simulink library "sm_worm_jack_lib"  (R2021b)
settings: Solver=VariableStepAuto  StartTime=0.0  StopTime=10.0  RelTol=1e-3
undefined symbols (not defined in the file or in its folder): Hand, Right, X, Y, Z
libraries: sm_lib x37, $bdroot x11, nesl_utility x8
(part 1 of 2)
settings Model: Creator=The MathWorks, Inc.  LastModifiedBy=The MathWorks, Inc.
settings SolverCC: AlgebraicLoopSolver=TrustRegion
settings DataIOCC: ReturnWorkspaceOutputs=off
settings DebuggingCC: SFMachineParentedDataDiag=warning  ArithmeticOperatorsInVariantConditions=warning
settings SFSimCC: SimUseLocalCustomCode=off  CustomCodeUndefinedFunction=UseInterfaceOnly
settings RTWCC: RTWUseLocalCustomCode=off
settings CodeAppCC: StateflowObjectComments=on

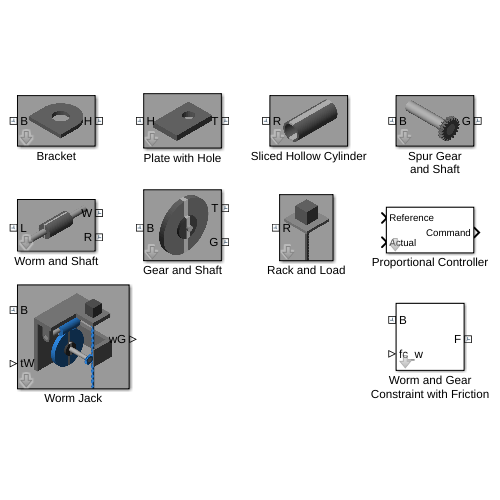
[thumbnail: Simulink's stored preview of the top-level diagram]
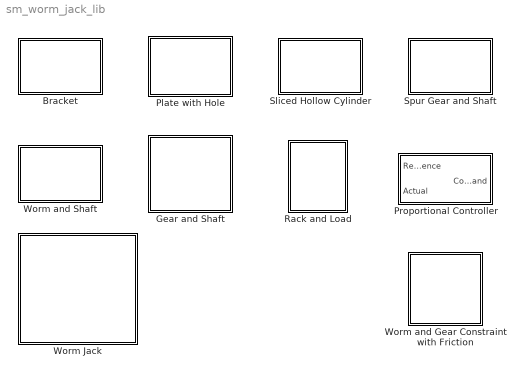
== system sm_worm_jack_lib ==
  Bracket : Subsystem  mask(Bracket){height=0.1, width=0.1, thickness=0.01, holeOffset=0.05, holeRadius=0.02, rho=2700, color=[0.5 0.5 0.5]}
      mask prompts: height "Height (m)"; width "Width (m)"; thickness "Thickness (m)"; holeOffset "Hole Offset (m)"; holeRadius "Hole Radius (m)"; rho "Density (kg/m^3)"; color "Color [r g b]"
      mask help:
      | This block models a bracket.
      |
      | Port B corresponds to the center point on the base face. Port H corresponds to the center of the hole.
      mask init:
      | points = 40;
      | 
      | y = height - 0.5*width;
      | 
      | outerVertices = ...
      |   [          0      0;...
      |      0.5*width      0;...
      |      0.5*width      y;...
      |      0.5*width height;...
      |     -0.5*width height;...
      |     -0.5*width      y;...
      |     -0.5*width      0;...
      |              0      0];
      | 
      | outer = simmechanics.demohelpers.round_corners(...
      |   outerVertices, [4 5], 0.5*width, points);
      | 
      | holeTheta = linspace(1.5*pi, -0.5*pi, points);
      | 
      | hole = [holeRadius*cos(holeTheta);...
      |         holeRadius*sin(holeTheta)+holeOffset]';
      | 
      | crossSection = [hole; outer];
      mask DialogControl Tab1 Prompt: Dimensions
      mask DialogControl Tab2 Prompt: Material Properties
      mask Display:
      | image(fullfile(matlabroot,'toolbox','physmod','sm','smdemos','worm_jack','images','sm_worm_jack_bracket.png'));
      | port_label('lconn',1,'B');
      | port_label('rconn',1,'H');
  Gear and Shaft : Subsystem  mask(Gear and Shaft){gearRadius=0.1, gearLength=0.02, shaftRadius=0.01, shaftLength=0.1, collarRadius=0.04, gearOffset=0.02, rhoGear=2700, rhoShaft=2700, rhoCollar=2700, gearColor=[0.5 0.5 0.5], shaftColor=[0.8 0.8 0.8], collarColor=[0.3 0.3 0.3], sliceColor=[0.9 0.9 0.9]}
      mask prompts: gearRadius "Gear Radius (m)"; gearLength "Gear Length (m)"; shaftRadius "Shaft Radius (m)"; shaftLength "Shaft Length (m)"; collarRadius "Collar Radius (m)"; gearOffset "Axial Offset (m)"; rhoGear "Gear Density (kg/m^3)"; rhoShaft "Shaft Density (kg/m^3)"; rhoCollar "Collar Density (kg/m^3)"; gearColor "Gear Color [r g b]"; shaftColor "Shaft Color [r g b]"; collarColor "Collar Color [r g b]"; sliceColor "Slice Color [r g b]"
      mask help:
      | This block models a gear mounted on a shaft with a collar. The gear, collar and shaft are concentric and the axial distance between the gear's midpoint and the shaft's midpoint can be adjusted.
      |
      | Ports B and T correspond to center points on the bottom and top faces of the shaft, respectively. Port G corresponds to the center of the gear.
      mask init:
      | offsetFromTop = 0.5*shaftLength-gearOffset;
      | 
      | sliceThickness = 0.4*collarRadius;
      mask DialogControl Tab1 Prompt: Dimensions
      mask DialogControl Tab2 Prompt: Material Properties
      mask Display:
      | image(fullfile(matlabroot,'toolbox','physmod','sm','smdemos','worm_jack','images','sm_worm_jack_gearshaft.png'));
      | port_label('lconn',1,'B');
      | port_label('rconn',1,'T');
      | port_label('rconn',2,'G');
  Plate with Hole : Subsystem  mask(Plate with Hole){height=0.15, width=0.1, thickness=0.02, holeRadius=0.02, holeOffset=0.1, rho=2700, color=[0.5 0.5 0.5]}
      mask prompts: height "Height (m)"; width "Width (m)"; thickness "Thickness (m)"; holeRadius "Hole Radius (m)"; holeOffset "Hole Offset (m)"; rho "Density (kg/m^3)"; color "Color [r g b]"
      mask help:
      | This block models a plate with a hole. The center of the hole is on the plate's longitudinal axis.
      |
      | Port H corresponds to the center of the hole. Port T corresponds to the center point on the top rear edge.
      mask init:
      | points = 40;
      | 
      | y = height - 0.5*width;
      | 
      | outer = ...
      |   [          0      0;...
      |      0.5*width      0;...
      |      0.5*width      y;...
      |      0.5*width height;...
      |     -0.5*width height;...
      |     -0.5*width      y;...
      |     -0.5*width      0;...
      |              0      0];
      | 
      | holeTheta = linspace(1.5*pi, -0.5*pi, points);
      | 
      | hole = [holeRadius*cos(holeTheta);...
      |         holeRadius*sin(holeTheta)+holeOffset]';
      | 
      | crossSection = [hole; outer];
      mask DialogControl Tab1 Prompt: Dimensions
      mask DialogControl Tab2 Prompt: Material Properties
      mask Display:
      | image(fullfile(matlabroot,'toolbox','physmod','sm','smdemos','worm_jack','images','sm_worm_jack_platehole.png'));
      | port_label('lconn',1,'H');
      | port_label('rconn',1,'T');
  Proportional Controller : Subsystem  mask(PID Controller){Kp=1}
      mask help:
      | This block models a proportional controller using Simulink blocks.
      |
      | This block takes in a reference signal and actual signal to calculate a control command.
  Rack and Load : Subsystem  mask(Rack and Load){rackWidth=0.01, rackBase=0.005, toothPitch=0.006, rackLength=0.3, plateWidth=0.1, plateThickness=0.01, loadWidth=0.05, rackRho=2700, plateRho=2700, loadRho=2700, rackColor=[0.5 0.5 0.5], plateColor=[0.7 0.7 0.7], loadColor=[0.5 0.5 0.5]}
      mask prompts: rackWidth "Rack Width (m)"; rackBase "Rack Base Thickness (m)"; toothPitch "Tooth Pitch (m)"; rackLength "Rack Length (m)"; plateWidth "Plate Width (m)"; plateThickness "Plate Thickness (m)"; loadWidth "Load Width (m)"; rackRho "Rack Density (kg/m^3)"; plateRho "Plate Density (kg/m^3)"; loadRho "Load Density (kg/m^3)"; rackColor "Rack Color [r g b]"; plateColor "Plate Color [r g b]"; loadColor "Load Color [r g b]"
      mask help:
      | This block models a rack that is attached to a load. The load consists of a brick which is carried on a rectangular plate.
      |
      | Port R corresponds to the center of the rack.
      mask init:
      | plateDimensions = [plateWidth plateWidth plateThickness];
      | loadDimensions  = loadWidth*[1 1 1];
      | 
      | numTeeth = ceil(rackLength/toothPitch);
      | 
      | rackCrossSection = ...
      |   simmechanics.demohelpers.rack_profile(toothPitch,numTeeth,rackBase);
      mask DialogControl TabVar1 Prompt: Dimensions
      mask DialogControl TabVar2 Prompt: Material Properties
      mask Display:
      | image(fullfile(matlabroot,'toolbox','physmod','sm','smdemos','worm_jack','images','sm_worm_jack_rackload.png'));
      | port_label('lconn',1,'R');
  Sliced Hollow Cylinder : Subsystem  mask(Sliced Hollow Cylinder){outerRadius=0.1, innerRadius=0.09, length=0.5, sliceThickness=0.06, rho=2700, mainColor=[0.5 0.5 0.5], sliceColor=[0.9 0.9 0.9]}
      mask prompts: outerRadius "Outer Radius (m)"; innerRadius "Inner Radius (m)"; length "Length (m)"; sliceThickness "Slice Thickness (m)"; rho "Density (kg/m^3)"; mainColor "Main Color [r g b]"; sliceColor "Slice Color [r g b]"
      mask help:
      | This block models a hollow cylinder where a slice of the cylinder can be set to a different color.
      |
      | Port R corresponds to the center of the cylinder.
      mask init:
      | points = 30;
      | 
      | outerTheta = acos(0.5*sliceThickness / outerRadius);
      | 
      | rightOuterThetaVect = linspace(  -outerTheta,      outerTheta, points);
      | leftOuterThetaVect  = linspace(pi-outerTheta,   pi+outerTheta, points);
      | topOuterThetaVect   = linspace(   outerTheta,   pi-outerTheta, points);
      | botOuterThetaVect   = linspace(pi+outerTheta, 2*pi-outerTheta, points);
      | 
      | if (sliceThickness > 2*innerRadius)
      |   % The slice is wider than the hole
      |   rightCrossSection = [outerRadius*cos(rightOuterThetaVect);...
      |                        outerRadius*sin(rightOuterThetaVect)]';
      |   leftCrossSection  = [outerRadius*cos(leftOuterThetaVect);...
      |                        outerRadius*sin(leftOuterThetaVect)]';
      | 
      |   topInnerThetaVect = linspace(pi, 0, points);
      |   botInnerThetaVect = linspace(0, -pi, points);
      |   
      |   topCrossSection = [...
      |     outerRadius*cos(topOuterThetaVect) -0.5*sliceThickness innerRadius*cos(topInnerThetaVect) 0.5*sliceThickness;...
      |     outerRadius*sin(topOuterThetaVect) 0 innerRadius*sin(topInnerThetaVect) 0]';
      |   
      |   botCrossSection = [...
      |     outerRadius*cos(botOuterThetaVect) 0.5*sliceThickness innerRadius*cos(botInnerThetaVect) -0.5*sliceThickness;...
      |     outerRadius*sin(botOuterThetaVect) 0 innerRadius*sin(botInnerThetaVect) 0]';
      | else
      |   % The slicer is narrower than the hole
      |   innerTheta = acos(0.5*sliceThickness / innerRadius);
      |   
      |   rightInnerThetaVect = linspace(   innerTheta,    -innerTheta, points);
      |   leftInnerThetaVect  = linspace(pi+innerTheta,  pi-innerTheta, points);
      |   topInnerThetaVect   = linspace(pi-innerTheta,     innerTheta, points);
      |   botInnerThetaVect   = linspace(  -innerTheta, -pi+innerTheta, points);
      |   
      |   rightCrossSection = [...
      |     outerRadius*cos(rightOuterThetaVect) innerRadius*cos(rightInnerThetaVect);...
      |     outerRadius*sin(rightOuterThetaVect) innerRadius*sin(rightInnerThetaVect)]';
      |   leftCrossSection  = [...
      |     outerRadius*cos(leftOuterThetaVect)  innerRadius*cos(leftInnerThetaVect);...
      |     outerRadius*sin(leftOuterThetaVect)  innerRadius*sin(leftInnerThetaVect)]';
      |   topCrossSection   = [...
      |     outerRadius*cos(topOuterThetaVect)   innerRadius*cos(topInnerThetaVect);...
      |     outerRadius*sin(topOuterThetaVect)   innerRadius*sin(topInnerThetaVect)]';
      |   botCrossSection   = [...
      |     outerRadius*cos(botOuterThetaVect)   innerRadius*cos(botInnerThetaVect);...
      |     outerRadius*sin(botOuterThetaVect)   innerRadius*sin(botInnerThetaVect)]';
      | end
      mask DialogControl Tab1 Prompt: Dimensions
      mask DialogControl Tab2 Prompt: Material Properties
      mask Display:
      | image(fullfile(matlabroot,'toolbox','physmod','sm','smdemos','worm_jack','images','sm_worm_jack_slicedhollowcylinder.png'));
      | port_label('lconn',1,'R');
  Spur Gear and Shaft : Subsystem  mask(Pinion Gear and Shaft){gearRadius=0.02, numTeeth=20, gearLength=0.01, shaftRadius=0.01, shaftLength=0.1, gearRho=2700, shaftRho=2700, gearColor=[0.5 0.5 0.5], shaftColor=[0.8 0.8 0.8]}
      mask prompts: gearRadius "Gear Radius (m)"; numTeeth "Number of Teeth"; gearLength "Gear Length (m)"; shaftRadius "Shaft Radius (m)"; shaftLength "Shaft Length (m)"; gearRho "Gear Density (kg/m^3)"; shaftRho "Shaft Density (kg/m^3)"; gearColor "Gear Color [r g b]"; shaftColor "Shaft Color [r g b]"
      mask help:
      | This block models a spur gear on a shaft. The gear and shaft are concentric and the number of gear teeth can be adjusted.
      |
      | Port B corresponds to the center point on the bottom face of the shaft. Port G corresponds to the center of the gear.
      mask init:
      | gearCrossSection = simmechanics.demohelpers.gear_profile(2*gearRadius,numTeeth);
      | gearCrossSection = [gearCrossSection; gearCrossSection(1,:)];
      | 
      | th = linspace(0,-2*pi,100)';
      | holeCrossSection = [shaftRadius*cos(th) shaftRadius*sin(th)];
      | 
      | gearCrossSection = [gearCrossSection; holeCrossSection];
      mask DialogControl TabVar1 Prompt: Dimensions
      mask DialogControl TabVar2 Prompt: Material Properties
      mask Display:
      | image(fullfile(matlabroot,'toolbox','physmod','sm','smdemos','worm_jack','images','sm_worm_jack_spurgearshaft.png'));
      | port_label('lconn',1,'B');
      | port_label('rconn',1,'G');
  Worm Jack : Subsystem  mask(Worm Drive Assembly){wormLeadAngle=10, wormRadius=0.025, wormLength=0.1, wormShaftLength=0.2, gearRadius=0.085, gearLength=0.02, gearShaftLength=0.1, collarRadius=0.03, shaftRadius=0.01, rackLength=0.4, pinionRadius=0.02, pinionTeeth=20, pinionShaftLength=0.1, loadWidth=0.05, plateThickness=0.02, wG_0=80, muK=0.5, muS=0.5, vth=1e-4, t_c=1e-6, wormRho=2700, gearRho=2700, shaftRho=2700, collarRho=2700, rackRho=2700, pinionRho=2700, housingRho=2700, boxRho=7800, wormColor=[0.2 0.6 1.0], gearColor=[0.2 0.6 1.0], shaftColor=[0.8 0.8 0.8], collarColor=[0.3 0.3 0.3], rackColor=[0.2 0.6 1.0], pinionColor=[0.2 0.6 1.0], housingColor=[0.6 0.6 0.6], boxColor=[0.4 0.4 0.4], sliceColor=[0.9 0.9 0.9]}
      mask prompts: wormLeadAngle "Worm Lead Angle (deg)"; wormRadius "Worm Radius (m)"; wormLength "Worm Length (m)"; wormShaftLength "Worm Shaft Length (m)"; gearRadius "Gear Radius (m)"; gearLength "Gear Length (m)"; gearShaftLength "Gear Shaft Length (m)"; collarRadius "Gear Collar Radius (m)"; shaftRadius "Shaft Radii (m)"; rackLength "Rack Length (m)"; pinionRadius "Pinion Radius (m)"; pinionTeeth "Pinion Teeth Number"; pinionShaftLength "Pinion Shaft Length (m)"; loadWidth "Load Width (m)"; plateThickness "Housing Plate Thickness (m)"; wG_0 "Initial Gear Revolute Velocity (deg/s)"; muK "Kinetic Friction Coefficient"; muS "Static Friction Coefficient"; vth "Velocity Threshold (m/s)"; t_c "Constraint Force Filter Constant (s)"; wormRho "Worm Density (kg/m^3)"; gearRho "Gear Density (kg/m^3)"; shaftRho "Shaft Density (kg/m^3)"; collarRho "Collar Density (kg/m^3)"; rackRho "Rack Density (kg/m^3)"; pinionRho "Pinion Density (kg/m^3)"; housingRho "Housing Density (kg/m^3)"; boxRho "Box Density (kg/m^3)"; wormColor "Worm Color [r g b]"; gearColor "Gear Color [r g b]"; shaftColor "Shaft Color [r g b]"; collarColor "Collar Color [r g b]"; rackColor "Rack Color [r g b]"; pinionColor "Pinion Color [r g b]"; housingColor "Housing Color [r g b]"; boxColor "Box Color [r g b]"; sliceColor "Slice Color [r g b]"
      mask help:
      | This block models a worm jack. The mechanism consists of a worm drive coupled to a rack and pinion.
      |
      | Port B corresponds to the center of the hole where the gear shaft is mounted.
      |
      | The input port tW specifies the torque input to the worm revolute joint. Output port wG corresponds to the angular velocity of the gear revolute joint.
      mask init:
      | wormShaftLength   = 2*gearRadius + 4*plateThickness;
      | pinionLength      = 0.5*pinionRadius;
      | rackWidth         = pinionLength;
      | rackBase          = 0.5*pinionLength;
      | toothPitch        = 2*pi*pinionRadius/pinionTeeth;
      | gearOffset        = 0.5*(gearShaftLength-3*gearLength);
      | housingHoleRadius = 1.1*shaftRadius;
      | gearSupHeight     = 2*gearRadius + 2*wormRadius + plateThickness;
      | bracketHoleOffset = plateThickness + wormRadius;
      | bracketHoleRadius = housingHoleRadius;
      | bracketWidth      = 4*shaftRadius;
      | bracketHeight     = bracketHoleOffset + 0.5*bracketWidth;
      | 
      | wormSupportDims = [wormShaftLength plateThickness gearShaftLength];
      | 
      | leftBracketOffset   = [ 0.5*(plateThickness-wormShaftLength) ...
      |                        -0.5*plateThickness                   ...
      |                         0.5*gearShaftLength-1.5*gearLength];
      |                       
      | rightBracketOffset  = [ 0.5*(wormShaftLength-plateThickness) ...
      |                        -0.5*plateThickness                   ...
      |                         0.5*gearShaftLength-1.5*gearLength];
      | 
      | % Rack Support
      | 
      | sidePlateYDim = (gearShaftLength+pinionShaftLength-1.5*plateThickness-0.5*pinionLength);
      | sidePlateDim  = [gearRadius sidePlateYDim plateThickness];
      | 
      | frontPlateYDim = (0.5*wormShaftLength-2*pinionRadius);
      | frontPlateDim  = [gearRadius frontPlateYDim plateThickness];
      | 
      | rackSupportOffset   = [0.5*(wormShaftLength-plateThickness) ...
      |                        0                                    ...
      |                        0.5*plateThickness];
      | 
      | guideDepth = pinionRadius;
      | guideWidth = pinionRadius;
      | 
      | guideCrossSection = [-0.5 *guideWidth 0;              ...
      |                       0.5 *guideWidth 0;              ...
      |                       0.5 *guideWidth guideDepth;     ...
      |                       0.25*guideWidth guideDepth;     ...
      |                       0.25*guideWidth 0.5*guideDepth; ...
      |                      -0.25*guideWidth 0.5*guideDepth; ...
      |                      -0.25*guideWidth guideDepth;     ...
      |                      -0.5 *guideWidth guideDepth];
      mask DialogControl Tab1 Prompt: Dimensions
      mask DialogControl Tab2 Prompt: Internal Mechanics
      mask DialogControl Tab3 Prompt: Material Properties
      mask Display:
      | image(fullfile(matlabroot,'toolbox','physmod','sm','smdemos','worm_jack','images','sm_worm_jack_wormjack.png'));
      | port_label('lconn',1,'B');
      | port_label('lconn',2,'tW');
      | port_label('rconn',1,'wG');
  Worm and Gear Constraint with Friction : Subsystem  mask(Worm and Gear Constraint with Friction){wormDirection=Right-Hand, wormLeadAngle=10, wormRadius=0.025, gearRadius=0.085, frictionToggle=on, muK=0.5, muS=0.5, vth=1e-4, t_c=1e-6}
      mask prompts: wormDirection "Worm Direction"; wormLeadAngle "Worm Lead Angle (deg)"; wormRadius "Worm Radius (m)"; gearRadius "Gear Radius (m)"; frictionToggle "Enable Friction"; muK "Kinetic Friction Coefficient"; muS "Static Friction Coefficient"; vth "Sliding Velocity Threshold (m/s)"; t_c "Constraint Force Filter Constant (s)"
      mask help:
      | This block models a Worm and Gear Constraint with friction. The worm rotates about the base z-axis and the gear rotates about the follower z-axis.
      |
      | Ports B and F are frame ports that represent the base and follower frames of the Worm and Gear Constraint block, respectively. The constraint force signal from the worm's revolute joint must be provided through port fc_w.
      mask init:
      | blockPath = gcb;
      | wgcPath = [blockPath '/Worm and Gear Constraint'];
      | 
      | if wormDirection == 1
      |     set_param(wgcPath,'WormDirection','RightHand');
      |     wormDirGain = 1;
      | else
      |     set_param(wgcPath,'WormDirection','LeftHand');
      |     wormDirGain = -1;
      | end
      | 
      | if frictionToggle
      |     frcGain = 1;
      | else
      |     frcGain = 0;
      | end
      mask TypeOptions wormDirection: Right-Hand | Left-Hand
      mask DialogControl Tab1 Prompt: Properties
      mask DialogControl Tab2 Prompt: Internal Mechanics
  Worm and Shaft : Subsystem  mask(Worm and Shaft){wormRadius=0.025, wormLength=0.1, shaftRadius=0.01, shaftLength=0.25, rhoWorm=2700, rhoShaft=2700, wormColor=[0.5 0.5 0.5], shaftColor=[0.8 0.8 0.8], sliceColor=[0.9 0.9 0.9]}
      mask prompts: wormRadius "Worm Radius (m)"; wormLength "Worm Length (m)"; shaftRadius "Shaft Radius (m)"; shaftLength "Shaft Length (m)"; rhoWorm "Worm Density (kg/m^3)"; rhoShaft "Shaft Density (kg/m^3)"; wormColor "Worm Color [r g b]"; shaftColor "Shaft Color [r g b]"; sliceColor "Slice Color [r g b]"
      mask help:
      | This block models a worm mounted on a shaft. The worm and shaft are concentric and the worm is axially located at the midpoint of the shaft.
      |
      | Ports L and R correspond to center points on the left and right faces of the shaft, respectively. Port W corresponds to the center of the worm.
      mask init:
      | sliceThickness = 0.2*wormRadius;
      mask DialogControl Tab1 Prompt: Dimensions
      mask DialogControl Tab2 Prompt: Material Properties
      mask Display:
      | image(fullfile(matlabroot,'toolbox','physmod','sm','smdemos','worm_jack','images','sm_worm_jack_wormshaft.png'));
      | port_label('lconn',1,'L');
      | port_label('rconn',1,'W');
      | port_label('rconn',2,'R');

== system sm_worm_jack_lib/Bracket ==
  Bracket : sm_lib/Body Elements/Extruded Solid  GraphicAmbientColor=[0.15 0.15 0.15 1.0]  BasedOnType=Density  CenterOfMass=[0 0 0]  CenterOfMassUnits=m  GraphicDiffuseColor=color  ExportConvexHullGeometry=off  ExtrusionCrossSection=crossSection  ExtrusionCrossSectionUnits=m  Density=rho  DensityUnits=kg/m^3  DoExposeReferenceFrame=on  GraphicEmissiveColor=[0.0 0.0 0.0 1.0]  ExportEntireGeometry=off  ExtrusionLength=thickness  ExtrusionLengthUnits=m  ExtrusionType=General  SerializedFrames=<Frames/>  MarkerShape=Sphere  MarkerSize=10  GraphicType=FromGeometry  InertiaType=CalculateFromGeometry  Mass=1  MassUnits=kg  MomentsOfInertia=[1 1 1]  MomentsOfInertiaUnits=kg*m^2  PolygonNumSides=3  GraphicOpacity=1.0  PolygonOuterRadius=1  PolygonOuterRadiusUnits=m  ProductsOfInertia=[1 1 1]  ProductsOfInertiaUnits=kg*m^2  GraphicShininess=75  GraphicSpecularColor=[0.5 0.5 0.5 1.0]  GraphicVisPropType=SimpleVisualProperties
  Hole xForm : sm_lib/Frames and Transforms/Rigid Transform  TranslationMethod=StandardAxis  TranslationStandardOffset=holeOffset  TranslationLengthUnit=m  TranslationStandardAxis=+Y  TranslationCartesianOffset=[0 0 0]  TranslationROffset=0  TranslationROffsetUnits=m  TranslationZOffset=0  TranslationZOffsetUnits=m  TranslationThetaOffset=0  TranslationThetaOffsetUnits=deg  RotationMethod=None  RotationAngleUnits=deg  RotationStandardAxis=+Y  RotationAngle=0.0  RotationArbitraryAxis=[0 0 1]  FollAlignAxisA=+X  BaseAlignAxisA=+Y  FollAlignAxisB=+Y  BaseAlignAxisB=+Z  RotationSequenceAxes=FollowerAxes  RotationSequence=XYX  RotationSequenceAngles=[0 0 0]  RotationSequenceAnglesUnits=deg  RotationMatrix=[1 0 0; 0 1 0; 0 0 1]
  B : PMIOPort  Side=Left
  H : PMIOPort  Port=2  Side=Right
  connections:
  B/RConn1 -- Hole xForm/LConn1 -- Bracket/RConn1
  H/RConn1 -- Hole xForm/RConn1

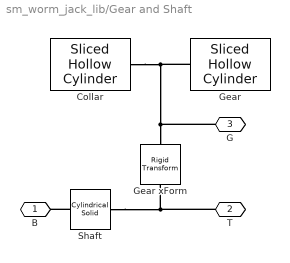
== system sm_worm_jack_lib/Gear and Shaft ==
  Collar : $bdroot/Sliced Hollow Cylinder  outerRadius=collarRadius  innerRadius=shaftRadius  length=2*gearLength  sliceThickness=sliceThickness  rho=rhoCollar  mainColor=collarColor  sliceColor=sliceColor
  Gear : $bdroot/Sliced Hollow Cylinder  outerRadius=gearRadius  innerRadius=collarRadius  length=gearLength  sliceThickness=sliceThickness  rho=rhoGear  mainColor=gearColor  sliceColor=sliceColor
  Gear xForm : sm_lib/Frames and Transforms/Rigid Transform  TranslationMethod=StandardAxis  TranslationStandardOffset=offsetFromTop  TranslationLengthUnit=m  TranslationStandardAxis=-Z  TranslationCartesianOffset=[0 0 0]  TranslationROffset=0  TranslationROffsetUnits=m  TranslationZOffset=0  TranslationZOffsetUnits=m  TranslationThetaOffset=0  TranslationThetaOffsetUnits=deg  RotationMethod=None  RotationAngleUnits=deg  RotationStandardAxis=+Z  RotationAngle=0.0  RotationArbitraryAxis=[0 0 1]  FollAlignAxisA=+X  BaseAlignAxisA=+Y  FollAlignAxisB=+Y  BaseAlignAxisB=+Z  RotationSequenceAxes=FollowerAxes  RotationSequence=XYX  RotationSequenceAngles=[0 0 0]  RotationSequenceAnglesUnits=deg  RotationMatrix=[1 0 0; 0 1 0; 0 0 1]
  Shaft : sm_lib/Body Elements/Cylindrical Solid  GraphicAmbientColor=[0.15 0.15 0.15 1.0]  BasedOnType=Density  CenterOfMass=[0 0 0]  CenterOfMassUnits=m  GraphicDiffuseColor=shaftColor  CylinderLength=shaftLength  CylinderLengthUnits=m  CylinderRadius=shaftRadius  CylinderRadiusUnits=m  Density=rhoShaft  DensityUnits=kg/m^3  DoExposeReferenceFrame=off  GraphicEmissiveColor=[0.0 0.0 0.0 1.0]  ExportEntireGeometry=off  SerializedFrames=<Frames><Frame><Id>Frame1</Id><Value><Name>T</Name><Origin><Source>GeometricFeature</Source><FeatureName>top surface</FeatureName></Origin><PrimaryAxis><DefinedDirection>+Z</DefinedDirection><Source>ReferenceFrame</Source><SourceDirection>+Z</SourceDirection><FeatureName></FeatureName></PrimaryAxis><SecondaryAxis><DefinedDirection>+X</DefinedDirection><Source>ReferenceFrame</Source><SourceDirection>+X</SourceDirection><FeatureName></FeatureName></SecondaryAxis></Value></Frame><Frame><Id>Frame2</Id><Value><Name>B</Name><Origin><Source>GeometricFeature</Source><FeatureName>bottom surface</FeatureName></Origin><PrimaryAxis><DefinedDirection>+Z</DefinedDirection><Source>ReferenceFrame</Source><SourceDirection>+Z</SourceDirection><FeatureName></FeatureName></PrimaryAxis><SecondaryAxis><DefinedDirection>+X</DefinedDirection><Source>ReferenceFrame</Source><SourceDirection>+X</SourceDirection><FeatureName></FeatureName></SecondaryAxis></Value></Frame></Frames>  MarkerShape=Sphere  MarkerSize=10  GraphicType=FromGeometry  InertiaType=CalculateFromGeometry  Mass=1  MassUnits=kg  MomentsOfInertia=[1 1 1]  MomentsOfInertiaUnits=kg*m^2  GraphicOpacity=1.0  ProductsOfInertia=[1 1 1]  ProductsOfInertiaUnits=kg*m^2  GraphicShininess=75  GraphicSpecularColor=[0.5 0.5 0.5 1.0]  GraphicVisPropType=SimpleVisualProperties
  B : PMIOPort  Side=Left
  T : PMIOPort  Port=2  Side=Right
  G : PMIOPort  Port=3  Side=Right
  connections:
  Gear/LConn1 -- Collar/LConn1 -- G/RConn1 -- Gear xForm/RConn1
  Shaft/LConn1 -- Gear xForm/LConn1 -- T/RConn1
  Shaft/RConn1 -- B/RConn1

== system sm_worm_jack_lib/Plate with Hole ==
  Hole xForm : sm_lib/Frames and Transforms/Rigid Transform  TranslationMethod=StandardAxis  TranslationStandardOffset=holeOffset  TranslationLengthUnit=m  TranslationStandardAxis=+Y  TranslationCartesianOffset=[0 0 0]  TranslationROffset=0  TranslationROffsetUnits=m  TranslationZOffset=0  TranslationZOffsetUnits=m  TranslationThetaOffset=0  TranslationThetaOffsetUnits=deg  RotationMethod=None  RotationAngleUnits=deg  RotationStandardAxis=+Y  RotationAngle=0.0  RotationArbitraryAxis=[0 0 1]  FollAlignAxisA=+X  BaseAlignAxisA=+Y  FollAlignAxisB=+Y  BaseAlignAxisB=+Z  RotationSequenceAxes=FollowerAxes  RotationSequence=XYX  RotationSequenceAngles=[0 0 0]  RotationSequenceAnglesUnits=deg  RotationMatrix=[1 0 0; 0 1 0; 0 0 1]
  Plate : sm_lib/Body Elements/Extruded Solid  GraphicAmbientColor=[0.15 0.15 0.15 1.0]  BasedOnType=Density  CenterOfMass=[0 0 0]  CenterOfMassUnits=m  GraphicDiffuseColor=color  ExportConvexHullGeometry=off  ExtrusionCrossSection=crossSection  ExtrusionCrossSectionUnits=m  Density=rho  DensityUnits=kg/m^3  DoExposeReferenceFrame=on  GraphicEmissiveColor=[0.0 0.0 0.0 1.0]  ExportEntireGeometry=off  ExtrusionLength=thickness  ExtrusionLengthUnits=m  ExtrusionType=General  SerializedFrames=<Frames><Frame><Id>Frame1</Id><Value><Name>T</Name><Origin><Source>GeometricFeature</Source><FeatureName>bottom curve 44</FeatureName></Origin><PrimaryAxis><DefinedDirection>+Z</DefinedDirection><Source>ReferenceFrame</Source><SourceDirection>+Z</SourceDirection><FeatureName></FeatureName></PrimaryAxis><SecondaryAxis><DefinedDirection>+X</DefinedDirection><Source>ReferenceFrame</Source><SourceDirection>+X</SourceDirection><FeatureName></FeatureName></SecondaryAxis></Value></Frame></Frames>  MarkerShape=Sphere  MarkerSize=10  GraphicType=FromGeometry  InertiaType=CalculateFromGeometry  Mass=1  MassUnits=kg  MomentsOfInertia=[1 1 1]  MomentsOfInertiaUnits=kg*m^2  PolygonNumSides=3  GraphicOpacity=1.0  PolygonOuterRadius=1  PolygonOuterRadiusUnits=m  ProductsOfInertia=[1 1 1]  ProductsOfInertiaUnits=kg*m^2  GraphicShininess=75  GraphicSpecularColor=[0.5 0.5 0.5 1.0]  GraphicVisPropType=SimpleVisualProperties
  H : PMIOPort  Side=Left
  T : PMIOPort  Port=2  Side=Right
  connections:
  T/RConn1 -- Plate/LConn1
  H/RConn1 -- Hole xForm/RConn1
  Hole xForm/LConn1 -- Plate/RConn1

== system sm_worm_jack_lib/Proportional Controller ==
  Reference : Inport
  Actual : Inport  Port=2
  Proportional Gain : Gain  Gain=Kp
  Sum : Sum  Inputs=+-|
  Command : Outport
  wires:
  Actual/1 -> Sum/2
  Reference/1 -> Sum/1
  Sum/1 -> Proportional Gain/1
  Proportional Gain/1 -> Command/1

== system sm_worm_jack_lib/Rack and Load ==
  Load : sm_lib/Body Elements/Brick Solid  GraphicAmbientColor=[0.15 0.15 0.15 1.0]  BasedOnType=Density  BrickDimensions=loadDimensions  BrickDimensionUnits=m  CenterOfMass=[0 0 0]  CenterOfMassUnits=m  GraphicDiffuseColor=loadColor  Density=loadRho  DensityUnits=kg/m^3  DoExposeReferenceFrame=off  GraphicEmissiveColor=[0.0 0.0 0.0 1.0]  ExportEntireGeometry=off  SerializedFrames=<Frames><Frame><Id>Frame1</Id><Value><Name>B</Name><Origin><Source>GeometricFeature</Source><FeatureName>-z surface</FeatureName></Origin><PrimaryAxis><DefinedDirection>+Z</DefinedDirection><Source>ReferenceFrame</Source><SourceDirection>+Z</SourceDirection><FeatureName></FeatureName></PrimaryAxis><SecondaryAxis><DefinedDirection>+X</DefinedDirection><Source>ReferenceFrame</Source><SourceDirection>+X</SourceDirection><FeatureName></FeatureName></SecondaryAxis></Value></Frame></Frames>  MarkerShape=Sphere  MarkerSize=10  GraphicType=FromGeometry  InertiaType=CalculateFromGeometry  Mass=1  MassUnits=kg  MomentsOfInertia=[1 1 1]  MomentsOfInertiaUnits=kg*m^2  GraphicOpacity=1.0  ProductsOfInertia=[1 1 1]  ProductsOfInertiaUnits=kg*m^2  GraphicShininess=75  GraphicSpecularColor=[0.5 0.5 0.5 1.0]  GraphicVisPropType=SimpleVisualProperties
  Plate : sm_lib/Body Elements/Brick Solid  GraphicAmbientColor=[0.15 0.15 0.15 1.0]  BasedOnType=Density  BrickDimensions=plateDimensions  BrickDimensionUnits=m  CenterOfMass=[0 0 0]  CenterOfMassUnits=m  GraphicDiffuseColor=plateColor  Density=plateRho  DensityUnits=kg/m^3  DoExposeReferenceFrame=off  GraphicEmissiveColor=[0.0 0.0 0.0 1.0]  ExportEntireGeometry=off  SerializedFrames=<Frames><Frame><Id>Frame1</Id><Value><Name>B</Name><Origin><Source>GeometricFeature</Source><FeatureName>-z surface</FeatureName></Origin><PrimaryAxis><DefinedDirection>+Z</DefinedDirection><Source>ReferenceFrame</Source><SourceDirection>+Z</SourceDirection><FeatureName></FeatureName></PrimaryAxis><SecondaryAxis><DefinedDirection>+X</DefinedDirection><Source>ReferenceFrame</Source><SourceDirection>+X</SourceDirection><FeatureName></FeatureName></SecondaryAxis></Value></Frame><Frame><Id>Frame2</Id><Value><Name>T</Name><Origin><Source>GeometricFeature</Source><FeatureName>+z surface</FeatureName></Origin><PrimaryAxis><DefinedDirection>+Z</DefinedDirection><Source>ReferenceFrame</Source><SourceDirection>+Z</SourceDirection><FeatureName></FeatureName></PrimaryAxis><SecondaryAxis><DefinedDirection>+X</DefinedDirection><Source>ReferenceFrame</Source><SourceDirection>+X</SourceDirection><FeatureName></FeatureName></SecondaryAxis></Value></Frame></Frames>  MarkerShape=Sphere  MarkerSize=10  GraphicType=FromGeometry  InertiaType=CalculateFromGeometry  Mass=1  MassUnits=kg  MomentsOfInertia=[1 1 1]  MomentsOfInertiaUnits=kg*m^2  GraphicOpacity=1.0  ProductsOfInertia=[1 1 1]  ProductsOfInertiaUnits=kg*m^2  GraphicShininess=75  GraphicSpecularColor=[0.5 0.5 0.5 1.0]  GraphicVisPropType=SimpleVisualProperties
  Rack : sm_lib/Body Elements/Extruded Solid  GraphicAmbientColor=[0.15 0.15 0.15 1.0]  BasedOnType=Density  CenterOfMass=[0 0 0]  CenterOfMassUnits=m  GraphicDiffuseColor=rackColor  ExportConvexHullGeometry=off  ExtrusionCrossSection=rackCrossSection  ExtrusionCrossSectionUnits=m  Density=rackRho  DensityUnits=kg/m^3  DoExposeReferenceFrame=off  GraphicEmissiveColor=[0.0 0.0 0.0 1.0]  ExportEntireGeometry=off  ExtrusionLength=rackWidth  ExtrusionLengthUnits=m  ExtrusionType=General  SerializedFrames=<Frames><Frame><Id>Frame1</Id><Value><Name>T</Name><Origin><Source>GeometricFeature</Source><FeatureName>side surface 1</FeatureName></Origin><PrimaryAxis><DefinedDirection>+Z</DefinedDirection><Source>ReferenceFrame</Source><SourceDirection>+X</SourceDirection><FeatureName></FeatureName></PrimaryAxis><SecondaryAxis><DefinedDirection>+Y</DefinedDirection><Source>ReferenceFrame</Source><SourceDirection>+Y</SourceDirection><FeatureName></FeatureName></SecondaryAxis></Value></Frame><Frame><Id>Frame2</Id><Value><Name>R</Name><Origin><Source>ReferenceFrame</Source><FeatureName></FeatureName></Origin><PrimaryAxis><DefinedDirection>+Z</DefinedDirection><Source>ReferenceFrame</Source><SourceDirection>+X</SourceDirection><FeatureName></FeatureName></PrimaryAxis><SecondaryAxis><DefinedDirection>+Y</DefinedDirection><Source>ReferenceFrame</Source><SourceDirection>+Y</SourceDirection><FeatureName></FeatureName></SecondaryAxis></Value></Frame></Frames>  MarkerShape=Sphere  MarkerSize=10  GraphicType=FromGeometry  InertiaType=CalculateFromGeometry  Mass=1  MassUnits=kg  MomentsOfInertia=[1 1 1]  MomentsOfInertiaUnits=kg*m^2  PolygonNumSides=3  GraphicOpacity=1.0  PolygonOuterRadius=1  PolygonOuterRadiusUnits=m  ProductsOfInertia=[1 1 1]  ProductsOfInertiaUnits=kg*m^2  GraphicShininess=75  GraphicSpecularColor=[0.5 0.5 0.5 1.0]  GraphicVisPropType=SimpleVisualProperties
  R : PMIOPort  Side=Left
  connections:
  Rack/RConn1 -- R/RConn1
  Load/LConn1 -- Plate/RConn1
  Plate/LConn1 -- Rack/LConn1

== system sm_worm_jack_lib/Sliced Hollow Cylinder ==
  Bottom : sm_lib/Body Elements/Extruded Solid  GraphicAmbientColor=[0.15 0.15 0.15 1.0]  BasedOnType=Density  CenterOfMass=[0 0 0]  CenterOfMassUnits=m  GraphicDiffuseColor=sliceColor  ExportConvexHullGeometry=off  ExtrusionCrossSection=botCrossSection  ExtrusionCrossSectionUnits=m  Density=rho  DensityUnits=kg/m^3  DoExposeReferenceFrame=on  GraphicEmissiveColor=[0.0 0.0 0.0 1.0]  ExportEntireGeometry=off  ExtrusionLength=length  ExtrusionLengthUnits=m  ExtrusionType=General  SerializedFrames=<Frames/>  MarkerShape=Sphere  MarkerSize=10  GraphicType=FromGeometry  InertiaType=CalculateFromGeometry  Mass=1  MassUnits=kg  MomentsOfInertia=[1 1 1]  MomentsOfInertiaUnits=kg*m^2  PolygonNumSides=3  GraphicOpacity=1.0  PolygonOuterRadius=1  PolygonOuterRadiusUnits=m  ProductsOfInertia=[1 1 1]  ProductsOfInertiaUnits=kg*m^2  GraphicShininess=75  GraphicSpecularColor=[0.5 0.5 0.5 1.0]  GraphicVisPropType=SimpleVisualProperties
  Left : sm_lib/Body Elements/Extruded Solid  GraphicAmbientColor=[0.15 0.15 0.15 1.0]  BasedOnType=Density  CenterOfMass=[0 0 0]  CenterOfMassUnits=m  GraphicDiffuseColor=mainColor  ExportConvexHullGeometry=off  ExtrusionCrossSection=leftCrossSection  ExtrusionCrossSectionUnits=m  Density=rho  DensityUnits=kg/m^3  DoExposeReferenceFrame=on  GraphicEmissiveColor=[0.0 0.0 0.0 1.0]  ExportEntireGeometry=off  ExtrusionLength=length  ExtrusionLengthUnits=m  ExtrusionType=General  SerializedFrames=<Frames/>  MarkerShape=Sphere  MarkerSize=10  GraphicType=FromGeometry  InertiaType=CalculateFromGeometry  Mass=1  MassUnits=kg  MomentsOfInertia=[1 1 1]  MomentsOfInertiaUnits=kg*m^2  PolygonNumSides=3  GraphicOpacity=1.0  PolygonOuterRadius=1  PolygonOuterRadiusUnits=m  ProductsOfInertia=[1 1 1]  ProductsOfInertiaUnits=kg*m^2  GraphicShininess=75  GraphicSpecularColor=[0.5 0.5 0.5 1.0]  GraphicVisPropType=SimpleVisualProperties
  Right : sm_lib/Body Elements/Extruded Solid  GraphicAmbientColor=[0.15 0.15 0.15 1.0]  BasedOnType=Density  CenterOfMass=[0 0 0]  CenterOfMassUnits=m  GraphicDiffuseColor=mainColor  ExportConvexHullGeometry=off  ExtrusionCrossSection=rightCrossSection  ExtrusionCrossSectionUnits=m  Density=rho  DensityUnits=kg/m^3  DoExposeReferenceFrame=on  GraphicEmissiveColor=[0.0 0.0 0.0 1.0]  ExportEntireGeometry=off  ExtrusionLength=length  ExtrusionLengthUnits=m  ExtrusionType=General  SerializedFrames=<Frames/>  MarkerShape=Sphere  MarkerSize=10  GraphicType=FromGeometry  InertiaType=CalculateFromGeometry  Mass=1  MassUnits=kg  MomentsOfInertia=[1 1 1]  MomentsOfInertiaUnits=kg*m^2  PolygonNumSides=3  GraphicOpacity=1.0  PolygonOuterRadius=1  PolygonOuterRadiusUnits=m  ProductsOfInertia=[1 1 1]  ProductsOfInertiaUnits=kg*m^2  GraphicShininess=75  GraphicSpecularColor=[0.5 0.5 0.5 1.0]  GraphicVisPropType=SimpleVisualProperties
  Top : sm_lib/Body Elements/Extruded Solid  GraphicAmbientColor=[0.15 0.15 0.15 1.0]  BasedOnType=Density  CenterOfMass=[0 0 0]  CenterOfMassUnits=m  GraphicDiffuseColor=sliceColor  ExportConvexHullGeometry=off  ExtrusionCrossSection=topCrossSection  ExtrusionCrossSectionUnits=m  Density=rho  DensityUnits=kg/m^3  DoExposeReferenceFrame=on  GraphicEmissiveColor=[0.0 0.0 0.0 1.0]  ExportEntireGeometry=off  ExtrusionLength=length  ExtrusionLengthUnits=m  ExtrusionType=General  SerializedFrames=<Frames/>  MarkerShape=Sphere  MarkerSize=10  GraphicType=FromGeometry  InertiaType=CalculateFromGeometry  Mass=1  MassUnits=kg  MomentsOfInertia=[1 1 1]  MomentsOfInertiaUnits=kg*m^2  PolygonNumSides=3  GraphicOpacity=1.0  PolygonOuterRadius=1  PolygonOuterRadiusUnits=m  ProductsOfInertia=[1 1 1]  ProductsOfInertiaUnits=kg*m^2  GraphicShininess=75  GraphicSpecularColor=[0.5 0.5 0.5 1.0]  GraphicVisPropType=SimpleVisualProperties
  R : PMIOPort  Side=Left
  connections:
  Left/RConn1 -- R/RConn1 -- Right/RConn1 -- Bottom/RConn1 -- Top/RConn1

== system sm_worm_jack_lib/Spur Gear and Shaft ==
  Gear : sm_lib/Body Elements/Extruded Solid  GraphicAmbientColor=[0.15 0.15 0.15 1.0]  BasedOnType=Density  CenterOfMass=[0 0 0]  CenterOfMassUnits=m  GraphicDiffuseColor=gearColor  ExportConvexHullGeometry=off  ExtrusionCrossSection=gearCrossSection  ExtrusionCrossSectionUnits=m  Density=gearRho  DensityUnits=kg/(m^3)  DoExposeReferenceFrame=off  GraphicEmissiveColor=[0.0 0.0 0.0 1.0]  ExportEntireGeometry=off  ExtrusionLength=gearLength  ExtrusionLengthUnits=m  ExtrusionType=General  SerializedFrames=<Frames><Frame><Id>Frame1</Id><Value><Name>T</Name><Origin><Source>GeometricFeature</Source><FeatureName>top surface</FeatureName></Origin><PrimaryAxis><DefinedDirection>+Z</DefinedDirection><Source>ReferenceFrame</Source><SourceDirection>+Z</SourceDirection><FeatureName></FeatureName></PrimaryAxis><SecondaryAxis><DefinedDirection>+X</DefinedDirection><Source>ReferenceFrame</Source><SourceDirection>+X</SourceDirection><FeatureName></FeatureName></SecondaryAxis></Value></Frame><Frame><Id>Frame2</Id><Value><Name>G</Name><Origin><Source>ReferenceFrame</Source><FeatureName></FeatureName></Origin><PrimaryAxis><DefinedDirection>+Z</DefinedDirection><Source>ReferenceFrame</Source><SourceDirection>+Z</SourceDirection><FeatureName></FeatureName></PrimaryAxis><SecondaryAxis><DefinedDirection>+X</DefinedDirection><Source>ReferenceFrame</Source><SourceDirection>+Y</SourceDirection><FeatureName></FeatureName></SecondaryAxis></Value></Frame></Frames>  MarkerShape=Sphere  MarkerSize=10  GraphicType=FromGeometry  InertiaType=CalculateFromGeometry  Mass=1  MassUnits=kg  MomentsOfInertia=[1 1 1]  MomentsOfInertiaUnits=kg*m^2  PolygonNumSides=3  GraphicOpacity=1.0  PolygonOuterRadius=1  PolygonOuterRadiusUnits=m  ProductsOfInertia=[0 0 0]  ProductsOfInertiaUnits=kg*m^2  GraphicShininess=75  GraphicSpecularColor=[0.5 0.5 0.5 1.0]  GraphicVisPropType=SimpleVisualProperties
  Shaft : sm_lib/Body Elements/Cylindrical Solid  GraphicAmbientColor=[0.15 0.15 0.15 1.0]  BasedOnType=Density  CenterOfMass=[0 0 0]  CenterOfMassUnits=m  GraphicDiffuseColor=shaftColor  CylinderLength=shaftLength  CylinderLengthUnits=m  CylinderRadius=shaftRadius  CylinderRadiusUnits=m  Density=shaftRho  DensityUnits=kg/m^3  DoExposeReferenceFrame=off  GraphicEmissiveColor=[0.0 0.0 0.0 1.0]  ExportEntireGeometry=off  SerializedFrames=<Frames><Frame><Id>Frame1</Id><Value><Name>B</Name><Origin><Source>GeometricFeature</Source><FeatureName>bottom surface</FeatureName></Origin><PrimaryAxis><DefinedDirection>+Z</DefinedDirection><Source>ReferenceFrame</Source><SourceDirection>+Z</SourceDirection><FeatureName></FeatureName></PrimaryAxis><SecondaryAxis><DefinedDirection>+X</DefinedDirection><Source>ReferenceFrame</Source><SourceDirection>+X</SourceDirection><FeatureName></FeatureName></SecondaryAxis></Value></Frame><Frame><Id>Frame2</Id><Value><Name>T</Name><Origin><Source>GeometricFeature</Source><FeatureName>top surface</FeatureName></Origin><PrimaryAxis><DefinedDirection>+Z</DefinedDirection><Source>ReferenceFrame</Source><SourceDirection>+Z</SourceDirection><FeatureName></FeatureName></PrimaryAxis><SecondaryAxis><DefinedDirection>+X</DefinedDirection><Source>ReferenceFrame</Source><SourceDirection>+X</SourceDirection><FeatureName></FeatureName></SecondaryAxis></Value></Frame></Frames>  MarkerShape=Sphere  MarkerSize=10  GraphicType=FromGeometry  InertiaType=CalculateFromGeometry  Mass=1  MassUnits=kg  MomentsOfInertia=[1 1 1]  MomentsOfInertiaUnits=kg*m^2  GraphicOpacity=1.0  ProductsOfInertia=[1 1 1]  ProductsOfInertiaUnits=kg*m^2  GraphicShininess=75  GraphicSpecularColor=[0.5 0.5 0.5 1.0]  GraphicVisPropType=SimpleVisualProperties
  B : PMIOPort  Side=Left
  G : PMIOPort  Port=2  Side=Right
  connections:
  Shaft/LConn1 -- B/RConn1
  Gear/LConn1 -- Shaft/RConn1
  G/RConn1 -- Gear/RConn1
